simulink model "ultra"  (R2020b)
settings: Solver=FixedStepDiscrete  StartTime=0.0  StopTime=10.0  FixedStep=0.0005  RelTol=1e-3  EnableMultiTasking=on
undefined symbols (not defined in the file): acc_calmax1, acc_calmax2, acc_calmin1, acc_calmin2, akemancanshu, bre, bre_calmax, bre_calmin, ecucoder_acal, I_AN01_5K1, I_AN03_5V, I_AN04_5V, kd, ki, kp, leftmax, O_SW06_HS1A, rightmax, T_add, T_del, tiaoshi, zhiling
libraries: ec5744lib x215, canmsglib x75, simulink x10
(part 5 of 7)

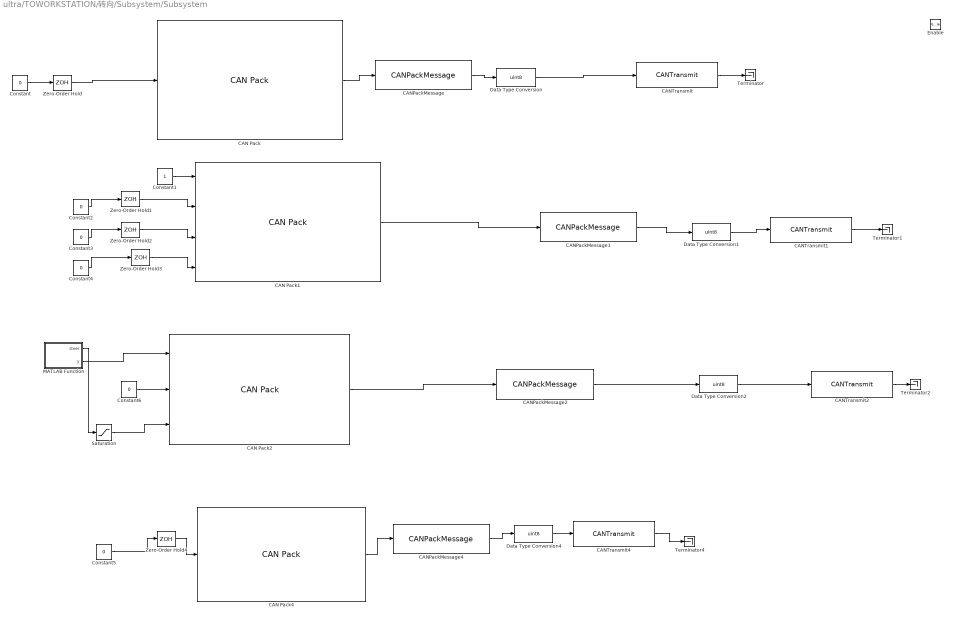
== system ultra/TOWORKSTATION/转向/Subsystem/Subsystem ==
  Enable : EnablePort
  CAN Pack : canmsglib/CAN Pack  CANdbFile=C:\Users\Liu keliang\Desktop\HRT2023\HRT23赛季刘科良\CANdbc\steering.dbc  MsgList=enable123  MsgName=enable123  MsgIDType=Standard (11-bit identifier)  MsgIdentifier=291  MsgLength=1  Remote=off  ApplyMinMax=off  BusOutput=off  SignalInfo={'enable123','0','8','LE','unsigned','Standard','0','1','0','0','255'}
      settings: SourceProductBaseCode=ME,XP,VN  DataFormat=CANdb specified signals
  CAN Pack1 : canmsglib/CAN Pack  CANdbFile=C:\Users\Liu keliang\Desktop\HRT2023\HRT23赛季刘科良\CANdbc\steering.dbc  MsgList=enable0  MsgName=enable0  MsgIDType=Standard (11-bit identifier)  MsgIdentifier=0  MsgLength=8  Remote=off  ApplyMinMax=off  BusOutput=off  SignalInfo={'enable_00','0','16','LE','unsigned','Standard','0','1','0','0','65535';'enable_00_Copy_1','16','16','LE','unsigned','Standard','0','1','0','0','65535';'enable_00_Copy_2','32','16','LE','unsigned','Standard','0','1','0','0','65535';'enable_00_Copy_3','48','16','LE','unsigned','Standard','0','1','0','0','65535'}
      settings: SourceProductBaseCode=ME,XP,VN  DataFormat=CANdb specified signals
  CAN Pack2 : canmsglib/CAN Pack  CANdbFile=C:\Users\Liu keliang\Desktop\HRT2023\HRT23赛季刘科良\CANdbc\steering.dbc  MsgList=enable401  MsgName=enable401  MsgIDType=Standard (11-bit identifier)  MsgIdentifier=1025  MsgLength=6  Remote=off  ApplyMinMax=off  BusOutput=off  SignalInfo={'enable401','0','8','LE','unsigned','Standard','0','1','0','0','255';'enable401_Copy_1','8','8','LE','unsigned','Standard','0','1','0','0','255';'enable401_Copy_2','16','32','LE','signed','Standard','0','1','0','-2147483648','2147483647'}
      settings: SourceProductBaseCode=ME,XP,VN  DataFormat=CANdb specified signals
  CAN Pack4 : canmsglib/CAN Pack  CANdbFile=C:\Users\Liu keliang\Desktop\HRT2023\HRT23赛季刘科良\CANdbc\steering.dbc  MsgList=enable80  MsgName=enable80  MsgIDType=Standard (11-bit identifier)  MsgIdentifier=128  MsgLength=1  Remote=off  ApplyMinMax=off  BusOutput=off  SignalInfo={'dingshi','0','8','LE','unsigned','Standard','0','1','0','0','255'}
      settings: SourceProductBaseCode=ME,XP,VN  DataFormat=CANdb specified signals
  CANPackMessage : ec5744lib/RapidECU_U4B/04CANCommunication/CANPackMessage  datalength=1  sampletime=-1
      settings: SourceProductName=ECUCoder for MPC5744
  CANPackMessage1 : ec5744lib/RapidECU_U4B/04CANCommunication/CANPackMessage  datalength=8  sampletime=-1
      settings: SourceProductName=ECUCoder for MPC5744
  CANPackMessage2 : ec5744lib/RapidECU_U4B/04CANCommunication/CANPackMessage  datalength=6  sampletime=-1
      settings: SourceProductName=ECUCoder for MPC5744
  CANPackMessage4 : ec5744lib/RapidECU_U4B/04CANCommunication/CANPackMessage  datalength=1  sampletime=-1
      settings: SourceProductName=ECUCoder for MPC5744
  CANTransmit : ec5744lib/RapidECU_U4B/04CANCommunication/CANTransmit  canmodule=1  canbuffer=15  canmessageid=hex2dec('123')  canmessagetype=Standard(11-bit ID)  datalength=1  sampletime=-1
      settings: SourceProductName=ECUCoder for MPC5744
  CANTransmit1 : ec5744lib/RapidECU_U4B/04CANCommunication/CANTransmit  canmodule=1  canbuffer=56  canmessageid=hex2dec('00')  canmessagetype=Standard(11-bit ID)  datalength=8  sampletime=-1
      settings: SourceProductName=ECUCoder for MPC5744
  CANTransmit2 : ec5744lib/RapidECU_U4B/04CANCommunication/CANTransmit  canmodule=1  canbuffer=57  canmessageid=hex2dec('401')  canmessagetype=Standard(11-bit ID)  datalength=6  sampletime=-1
      settings: SourceProductName=ECUCoder for MPC5744
  CANTransmit4 : ec5744lib/RapidECU_U4B/04CANCommunication/CANTransmit  canmodule=1  canbuffer=58  canmessageid=hex2dec('80')  canmessagetype=Standard(11-bit ID)  datalength=1  sampletime=-1
      settings: SourceProductName=ECUCoder for MPC5744
  Constant : Constant  Value=0  SampleTime=-1
  Constant1 : Constant  SampleTime=-1
  Constant{2..4,6} (4 alike) : Constant  Value=0
  Constant5 : Constant  Value=0  SampleTime=-1
  Data Type Conversion{,1..2,4} (4 alike) : DataTypeConversion  OutDataTypeStr=uint8
  MATLAB Function : MATLAB Function  TreatAsAtomicUnit=on
  Saturation : Saturate  UpperLimit=758000  LowerLimit=605000
  Terminator{,1..2,4} (4 alike) : Terminator
  Zero-Order Hold{,1..4} (5 alike) : ZeroOrderHold  SampleTime=-1
  wires:
  CANTransmit/1 -> Terminator/1
  Zero-Order Hold2/1 -> CAN Pack1/3
  MATLAB Function/2(y) -> CAN Pack2/1
  CAN Pack1/1 -> CANPackMessage1/1
  CANTransmit2/1 -> Terminator2/1
  CANPackMessage4/1 -> Data Type Conversion4/1
  CAN Pack2/1 -> CANPackMessage2/1
  CANTransmit1/1 -> Terminator1/1
  Constant/1 -> Zero-Order Hold/1
  Data Type Conversion1/1 -> CANTransmit1/1
  Constant6/1 -> CAN Pack2/2
  CANTransmit4/1 -> Terminator4/1
  Data Type Conversion/1 -> CANTransmit/1
  Zero-Order Hold/1 -> CAN Pack/1
  CANPackMessage2/1 -> Data Type Conversion2/1
  CANPackMessage/1 -> Data Type Conversion/1
  Data Type Conversion4/1 -> CANTransmit4/1
  Constant4/1 -> Zero-Order Hold3/1
  CAN Pack/1 -> CANPackMessage/1
  CANPackMessage1/1 -> Data Type Conversion1/1
  Constant5/1 -> Zero-Order Hold4/1
  CAN Pack4/1 -> CANPackMessage4/1
  Constant3/1 -> Zero-Order Hold2/1
  Constant2/1 -> Zero-Order Hold1/1
  Constant1/1 -> CAN Pack1/1
  Zero-Order Hold4/1 -> CAN Pack4/1
  MATLAB Function/1(steer) -> Saturation/1
  Zero-Order Hold1/1 -> CAN Pack1/2
  Data Type Conversion2/1 -> CANTransmit2/1
  Zero-Order Hold3/1 -> CAN Pack1/4
  Saturation/1 -> CAN Pack2/3

== system ultra/TOWORKSTATION/转向/Subsystem/Subsystem1 ==
  y1 : Inport
  y2 : Inport  Port=2
  Enable : EnablePort
  CAN Pack5 : canmsglib/CAN Pack  CANdbFile=C:\Users\Liu keliang\Desktop\HRT2023\HRT23赛季刘科良\CANdbc\zhuanxiangresetting.dbc  MsgList=reseting  MsgName=reseting  MsgIDType=Standard (11-bit identifier)  MsgIdentifier=1537  MsgLength=8  Remote=off  ApplyMinMax=off  BusOutput=off  SignalInfo={'reseting1','0','32','LE','unsigned','Standard','0','1','0','-Inf','Inf';'reseting2','32','32','LE','unsigned','Standard','0','1','0','-Inf','Inf'}
      settings: SourceProductBaseCode=ME,XP,VN  DataFormat=CANdb specified signals
  CANPackMessage3 : ec5744lib/RapidECU_U4B/04CANCommunication/CANPackMessage  datalength=8  sampletime=-1
      settings: SourceProductName=ECUCoder for MPC5744
  CANTransmit3 : ec5744lib/RapidECU_U4B/04CANCommunication/CANTransmit  canmodule=1  canbuffer=61  canmessageid=hex2dec('601')  canmessagetype=Standard(11-bit ID)  datalength=8  sampletime=-1
      settings: SourceProductName=ECUCoder for MPC5744
  Data Type Conversion3 : DataTypeConversion  OutDataTypeStr=uint8
  Terminator3 : Terminator
  wires:
  CAN Pack5/1 -> CANPackMessage3/1
  y1/1 -> CAN Pack5/1
  CANTransmit3/1 -> Terminator3/1
  Data Type Conversion3/1 -> CANTransmit3/1
  CANPackMessage3/1 -> Data Type Conversion3/1
  y2/1 -> CAN Pack5/2

== system ultra/TX控制器/扭矩/TEST/Subsystem ==
  Enable : EnablePort
  CAN Pack1 : canmsglib/CAN Pack  CANdbFile=C:\Users\Liu keliang\Desktop\HRT2023\HRT23赛季刘科良\CANdbc\TEST.dbc  MsgList=TEST  MsgName=TEST  MsgIDType=Standard (11-bit identifier)  MsgIdentifier=153  MsgLength=5  Remote=off  ApplyMinMax=off  BusOutput=off  SignalInfo={'M','16','8','LE','signed','Standard','0','1','0','-Inf','Inf';'X2D','32','8','LE','signed','Standard','0','1','0','-Inf','Inf';'a','0','8','LE','signed','Standard','0','1','0','-Inf','Inf';'deltv','8','8','LE','signed','Standard','0','1','0','-Inf','Inf';'niuju','24','8','LE','signed','Standard','0','1','0','-Inf','Inf'}
      settings: SourceProductBaseCode=ME,XP,VN  DataFormat=CANdb specified signals
  CANPackMessage1 : ec5744lib/RapidECU_U4B/04CANCommunication/CANPackMessage  datalength=5  sampletime=-1
      settings: SourceProductName=ECUCoder for MPC5744
  CANTransmit : ec5744lib/RapidECU_U4B/04CANCommunication/CANTransmit  canmodule=0  canbuffer=63  canmessageid=hex2dec('99')  canmessagetype=Standard(11-bit ID)  datalength=5  sampletime=-1
      settings: SourceProductName=ECUCoder for MPC5744
  Data Store Read : DataStoreRead  DataStoreName=a
  Data Store Read1 : DataStoreRead  DataStoreName=ve
  Data Store Read2 : DataStoreRead  DataStoreName=M
  Data Store Read3 : DataStoreRead  DataStoreName=acc
  Data Store Read4 : DataStoreRead  DataStoreName=dianji_velcoity_zuoqian
  Data Type Conversion1 : DataTypeConversion  OutDataTypeStr=uint8
  Terminator : Terminator
  wires:
  Data Store Read4/1 -> CAN Pack1/1
  CANTransmit/1 -> Terminator/1
  Data Store Read3/1 -> CAN Pack1/3
  CANPackMessage1/1 -> Data Type Conversion1/1
  Data Store Read2/1 -> CAN Pack1/5
  Data Type Conversion1/1 -> CANTransmit/1
  Data Store Read1/1 -> CAN Pack1/4
  Data Store Read/1 -> CAN Pack1/2
  CAN Pack1/1 -> CANPackMessage1/1

== system ultra/run/analog_input/无人意图转译/无人 ==
  Data Store Read : DataStoreRead  DataStoreName=match_model
  Data Store Write : DataStoreWrite  DataStoreName=escmax
  MATLAB Function3 : MATLAB Function  TreatAsAtomicUnit=on
  Max : MinMax  Function=max  Inputs=4
  Subsystem1 : Subsystem
  右前油压 : DataStoreWrite  DataStoreName=oral_pressure_rightfront
  右后油压 : DataStoreWrite  DataStoreName=oral_pressure_rightbehind
  左前油压 : DataStoreWrite  DataStoreName=oral_pressure_leftfront
  左后油压 : DataStoreWrite  DataStoreName=oral_pressure_leftbehind
  是否无人 : DataStoreWrite  DataStoreName=isdriveless
  期望加速度 : DataStoreWrite  DataStoreName=acc_expired
  期望纵向加速度 : Outport
  wires:
  Subsystem1/1(期望纵向加速度) -> 期望纵向加速度/1, 期望加速度/1
  Data Store Read/1 -> MATLAB Function3/1(u)
  MATLAB Function3/1(y) -> 是否无人/1
  Subsystem1/2(输出左前油压) -> Max/1, 左前油压/1
  Subsystem1/4(输出左后油压2) -> Max/3, 左后油压/1
  Subsystem1/3(输出右前油压1) -> Max/2, 右前油压/1
  Subsystem1/5(输出右后油压3) -> Max/4, 右后油压/1
  Max/1 -> Data Store Write/1

== system ultra/run/analog_input/有人/Subsystem ==
  AnalogInput : ec5744lib/RapidECU_U4B/01BasicInput/AnalogInput  channel=52:I_AN03_5V  sampletime=-1
      settings: SourceProductName=ECUCoder for MPC5744
  AnalogInput1 : ec5744lib/RapidECU_U4B/01BasicInput/AnalogInput  channel=53:I_AN04_5V  sampletime=-1
      settings: SourceProductName=ECUCoder for MPC5744
  AnalogInput2 : ec5744lib/RapidECU_U4B/01BasicInput/AnalogInput  channel=34:I_AN01_5K1  sampletime=-1
      settings: SourceProductName=ECUCoder for MPC5744
  Data Type Conversion : DataTypeConversion  OutDataTypeStr=double
  ECCalVar1 : Constant  InitFcn=ecucoder_acal;  Value=acc_calmax1  OutDataTypeStr=double  SampleTime=-1
  ECCalVar2 : Constant  InitFcn=ecucoder_acal;  Value=acc_calmin1  OutDataTypeStr=double  SampleTime=-1
  ECCalVar3 : Constant  InitFcn=ecucoder_acal;  Value=acc_calmax2  OutDataTypeStr=double  SampleTime=-1
  ECCalVar4 : Constant  InitFcn=ecucoder_acal;  Value=acc_calmin2  OutDataTypeStr=double  SampleTime=-1
  ECCalVar5 : Constant  InitFcn=ecucoder_acal;  Value=bre_calmax  OutDataTypeStr=double  SampleTime=-1
  ECCalVar6 : Constant  InitFcn=ecucoder_acal;  Value=bre_calmin  OutDataTypeStr=double  SampleTime=-1
  ECCalVar7 : Constant  InitFcn=ecucoder_acal;  Value=bre  OutDataTypeStr=double  SampleTime=-1
  FRAMEnable : ec5744lib/RapidECU_U4B/12EEModule/FRAMEnable  Commented=on  framenable=off
      settings: SourceProductName=ECUCoder for MPC5744
  MATLAB Function : MATLAB Function  TreatAsAtomicUnit=on
  MATLAB Function1 : MATLAB Function  TreatAsAtomicUnit=on
  MATLAB Function2 : MATLAB Function  TreatAsAtomicUnit=on
  MATLAB Function5 : MATLAB Function  TreatAsAtomicUnit=on
  MeaModule1 : ec5744lib/RapidECU_U4B/07Calibration/MeaModule  signal=acc_ori_line1
      settings: SourceProductName=ECUCoder for MPC5744
  MeaModule2 : ec5744lib/RapidECU_U4B/07Calibration/MeaModule  signal=acc_ori_line2
      settings: SourceProductName=ECUCoder for MPC5744
  MeaModule3 : ec5744lib/RapidECU_U4B/07Calibration/MeaModule  signal=guiyi
      settings: SourceProductName=ECUCoder for MPC5744
  MeaModule5 : ec5744lib/RapidECU_U4B/07Calibration/MeaModule  signal=bre_ori_sig
      settings: SourceProductName=ECUCoder for MPC5744
  MeaModule6 : ec5744lib/RapidECU_U4B/07Calibration/MeaModule  signal=acc_result2
      settings: SourceProductName=ECUCoder for MPC5744
  MeaModule8 : ec5744lib/RapidECU_U4B/07Calibration/MeaModule  signal=acc_result1
      settings: SourceProductName=ECUCoder for MPC5744
  MeaModule9 : ec5744lib/RapidECU_U4B/07Calibration/MeaModule  signal=bre_result
      settings: SourceProductName=ECUCoder for MPC5744
  Subsystem : Subsystem  Commented=on
  Subsystem1 : Subsystem  Commented=on
  无人制动标志位 : DataStoreRead  DataStoreName=wurenzhidongdeng
  acc : Outport
  bre : Outport  Port=2
  wires:
  AnalogInput/1 -> MeaModule1/1
  MeaModule8/1 -> MATLAB Function5/1(acc_fin_sig1)
  AnalogInput2/1 -> MeaModule5/1
  MeaModule5/1 -> MATLAB Function1/1(u)
  AnalogInput1/1 -> MeaModule2/1
  MeaModule1/1 -> MATLAB Function/1(u)
  MeaModule2/1 -> MATLAB Function2/1(u)
  MeaModule9/1 -> bre/1, MATLAB Function5/3(bre_ori_sig)
  ECCalVar3/1 -> MATLAB Function2/3(max)
  MATLAB Function2/1(y) -> MeaModule6/1
  ECCalVar1/1 -> MATLAB Function/3(max)
  ECCalVar4/1 -> MATLAB Function2/2(min)
  MATLAB Function/1(y) -> MeaModule8/1
  ECCalVar2/1 -> MATLAB Function/2(min)
  Subsystem1/1(y) -> Subsystem/Enable
  MeaModule6/1 -> Data Type Conversion/1
  Data Type Conversion/1 -> MATLAB Function5/2(acc_fin_sig2)
  ECCalVar6/1 -> MATLAB Function1/2(min)
  ECCalVar5/1 -> MATLAB Function1/3(max)
  MATLAB Function5/1(y) -> MeaModule3/1
  MeaModule3/1 -> acc/1
  ECCalVar7/1 -> MATLAB Function5/4(bre)
  无人制动标志位/1 -> MeaModule9/1

== system ultra/run/analog_input/有人/Subsystem1 ==
  note: 标定
  acc_signal : Inport
  Constant : Constant  Value=35
  Data Store Read : DataStoreRead  DataStoreName=V_Kalman
  Data Type Conversion : DataTypeConversion  OutMin=[0]  OutMax=[1]  OutDataTypeStr=double
  Divide1 : Product  Inputs=**  OutDataTypeStr=uint16
  ECCalVar : Constant  InitFcn=ecucoder_acal;  Value=T_add  OutDataTypeStr=Inherit: Inherit via back propagation  SampleTime=-1
  ECCalVar1 : Constant  InitFcn=ecucoder_acal;  Value=T_del  OutDataTypeStr=Inherit: Inherit via back propagation  SampleTime=-1
  ECCalVar2 : Constant  InitFcn=ecucoder_acal;  Value=zhiling  OutDataTypeStr=Inherit: Inherit via back propagation  SampleTime=-1
  MATLAB Function : MATLAB Function  TreatAsAtomicUnit=on
  MATLAB Function1 : MATLAB Function  TreatAsAtomicUnit=on
  Saturation3 : Saturate  UpperLimit=2100  LowerLimit=0
  Saturation4 : Saturate  UpperLimit=1  LowerLimit=0
  Sum : Sum  Inputs=|++-
  Sum1 : Sum  Inputs=+--
  TP : Outport
  wires:
  Data Type Conversion/1 -> Saturation4/1
  acc_signal/1 -> Data Type Conversion/1
  Saturation4/1 -> Divide1/2
  Sum/1 -> Divide1/1
  ECCalVar1/1 -> Sum/3
  ECCalVar/1 -> Sum/1
  Saturation3/1 -> Sum/2
  Data Store Read/1 -> MATLAB Function/1(v)
  MATLAB Function/1(T) -> Saturation3/1
  Divide1/1 -> Sum1/1
  Constant/1 -> Sum1/2
  Sum1/1 -> MATLAB Function1/1(T)
  MATLAB Function1/1(TP) -> TP/1
  ECCalVar2/1 -> Sum1/3

== system ultra/run/ctrl/Subsystem1/control_strategy ==
  TP : Inport
  Data Store Read1 : DataStoreRead  DataStoreName=workstation_steering
  Data Store Read2 : DataStoreRead  DataStoreName=slipyouhou
  Data Store Read4 : DataStoreRead  DataStoreName=workstation_steering
  Data Store Read5 : DataStoreRead  DataStoreName=slipzuohou
  Data Store Read6 : DataStoreRead  DataStoreName=slipyuoqian
  Data Store Read7 : DataStoreRead  DataStoreName=slipzuoqian
  E,H : MATLAB Function  Commented=on  TreatAsAtomicUnit=on
  MATLAB Function : MATLAB Function  Commented=on  TreatAsAtomicUnit=on
  MATLAB Function1 : MATLAB Function  TreatAsAtomicUnit=on
  MATLAB Function2 : MATLAB Function  Commented=on  TreatAsAtomicUnit=on
  MATLAB Function3 : MATLAB Function  TreatAsAtomicUnit=on
  MPC : MATLAB Function  Commented=on  TreatAsAtomicUnit=on
  Subsystem : Subsystem  Commented=on
  Switch{,1..3} (4 alike) : Switch  Criteria=u2 > Threshold
  差速 : Subsystem
  滑模控制 : MATLAB Function  TreatAsAtomicUnit=on
  限滑 : Subsystem
  youhou : Outport
  youqian : Outport  Port=2
  zuohou : Outport  Port=3
  zuoqian : Outport  Port=4
  wires:
  TP/1 -> 差速/1(u), 限滑/1(In1)
  Data Store Read4/1 -> MATLAB Function1/1(angle)
  MATLAB Function1/1(y) -> Switch2/2, Switch3/2, Switch1/2, Switch/2
  限滑/1(youhou) -> Switch/3
  限滑/2(youqian) -> Switch1/3
  限滑/3(zuohou) -> Switch2/3
  限滑/4(zuoqian) -> Switch3/3
  MATLAB Function2/1(A) -> E,H/1(A)
  MATLAB Function2/2(B) -> E,H/2(B)
  MATLAB Function2/3(Q) -> E,H/3(Q)
  MATLAB Function2/4(R) -> E,H/4(R)
  MATLAB Function2/5(F) -> E,H/5(F)
  MATLAB Function2/6(N) -> E,H/6(N)
  差速/1(youhou) -> Switch/1
  差速/2(youqian) -> Switch1/1
  差速/3(zuohou) -> Switch2/1
  差速/4(zuoqian) -> Switch3/1
  Data Store Read1/1 -> MATLAB Function3/1(angle)
  MATLAB Function3/1(y) -> 差速/Enable
  Data Store Read7/1 -> 滑模控制/1(slip_ratio_fl)
  Switch/1 -> 滑模控制/8(driver_torque_cmd_rr)
  Data Store Read2/1 -> 滑模控制/4(slip_ratio_rr)
  Data Store Read6/1 -> 滑模控制/2(slip_ratio_fr)
  Switch3/1 -> 滑模控制/5(driver_torque_cmd_fl)
  Data Store Read5/1 -> 滑模控制/3(slip_ratio_rl)
  Switch1/1 -> 滑模控制/6(driver_torque_cmd_fr)
  Switch2/1 -> 滑模控制/7(driver_torque_cmd_rl)
  滑模控制/4(torque_cmd_rr) -> youhou/1
  滑模控制/2(torque_cmd_fr) -> youqian/1
  滑模控制/3(torque_cmd_rl) -> zuohou/1
  滑模控制/1(torque_cmd_fl) -> zuoqian/1

== system ultra/RX/工作站/Subsystem1/Subsystem1/Subsystem ==
  ID : Inport
  msg : Inport  Port=2
  CAN Unpack : canmsglib/CAN Unpack  CANdbFile=C:\Users\Liu keliang\Desktop\HRT2023\HRT23赛季刘科良\CANdbc\INSWORKSTATION.dbc  MsgList=ins  MsgName=ins  MsgIDType=Standard (11-bit identifier)  MsgIdentifier=33  MsgLength=8  SignalInfo={'Vx','32','16','LE','unsigned','Standard','0','1','0','0','65535';'Vy','48','16','LE','unsigned','Standard','0','1','0','0','65535';'ax','0','8','LE','signed','Standard','0','1','0','-128','127';'ay','8','16','LE','signed','Standard','0','1','0','-32768','32767';'az','24','8','LE','signed','Standard','0','1','0','-128','127'}  IDPort=off  TimestampPort=off  ErrorPort=off  RemotePort=off  LengthPort=off  StatusPort=off  ApplyMinMax=off
      settings: SourceProductBaseCode=ME,XP,VN  DataFormat=CANdb specified signals
  CANUnPackMessage : ec5744lib/RapidECU_U4B/04CANCommunication/CANUnPackMessage  datalength=8  canmessagetype=Standard(11-bit ID)  sampletime=-1
      settings: SourceProductName=ECUCoder for MPC5744
  Data Store Write : DataStoreWrite  DataStoreName=guandaovy
  wires:
  msg/1 -> CANUnPackMessage/2
  CANUnPackMessage/1 -> CAN Unpack/1
  ID/1 -> CANUnPackMessage/1
  CAN Unpack/2 -> Data Store Write/1

== system ultra/RX/工作站/Subsystem3/Subsystem/Subsystem ==
  Data Store Read : DataStoreRead  DataStoreName=CANOK_20
  Delay : Delay  DelayLength=1
  Delay1 : Delay
  Delay10 : Delay  DelayLength=11
  Delay11 : Delay  DelayLength=12
  Delay12 : Delay  DelayLength=13
  Delay13 : Delay  DelayLength=14
  Delay14 : Delay  DelayLength=15
  Delay15 : Delay  DelayLength=16
  Delay16 : Delay  DelayLength=17
  Delay17 : Delay  DelayLength=25
  Delay18 : Delay  DelayLength=18
  Delay19 : Delay  DelayLength=19
  Delay2 : Delay  DelayLength=3
  Delay20 : Delay  DelayLength=20
  Delay21 : Delay  DelayLength=21
  Delay22 : Delay  DelayLength=22
  Delay23 : Delay  DelayLength=26
  Delay24 : Delay  DelayLength=24
  Delay25 : Delay  DelayLength=27
  Delay3 : Delay  DelayLength=4
  Delay4 : Delay  DelayLength=5
  Delay5 : Delay  DelayLength=6
  Delay6 : Delay  DelayLength=7
  Delay7 : Delay  DelayLength=8
  Delay8 : Delay  DelayLength=9
  Delay9 : Delay  DelayLength=10
  OR : Logic  Operator=OR  Inputs=27  IconShape=distinctive  AllPortsSameDT=off  OutDataTypeStr=boolean
  Out1 : Outport
  wires:
  Delay2/1 -> OR/2
  Delay/1 -> OR/4
  Data Store Read/1 -> Delay23/1, Delay25/1, Delay17/1, Delay24/1, Delay22/1, Delay21/1, Delay20/1, Delay19/1, Delay18/1, Delay16/1, Delay15/1, Delay14/1, Delay13/1, Delay12/1, Delay11/1, Delay10/1, Delay8/1, Delay6/1, Delay5/1, Delay7/1, Delay9/1, OR/5, Delay3/1, Delay2/1, Delay1/1, Delay/1, Delay4/1
  Delay5/1 -> OR/7
  Delay1/1 -> OR/3
  Delay9/1 -> OR/11
  Delay7/1 -> OR/9
  Delay3/1 -> OR/1
  Delay8/1 -> OR/8
  Delay6/1 -> OR/6
  Delay4/1 -> OR/10
  OR/1 -> Out1/1
  Delay10/1 -> OR/12
  Delay11/1 -> OR/13
  Delay12/1 -> OR/14
  Delay13/1 -> OR/15
  Delay14/1 -> OR/16
  Delay15/1 -> OR/17
  Delay16/1 -> OR/18
  Delay18/1 -> OR/19
  Delay19/1 -> OR/20
  Delay20/1 -> OR/21
  Delay21/1 -> OR/22
  Delay22/1 -> OR/23
  Delay24/1 -> OR/24
  Delay17/1 -> OR/25
  Delay23/1 -> OR/27
  Delay25/1 -> OR/26

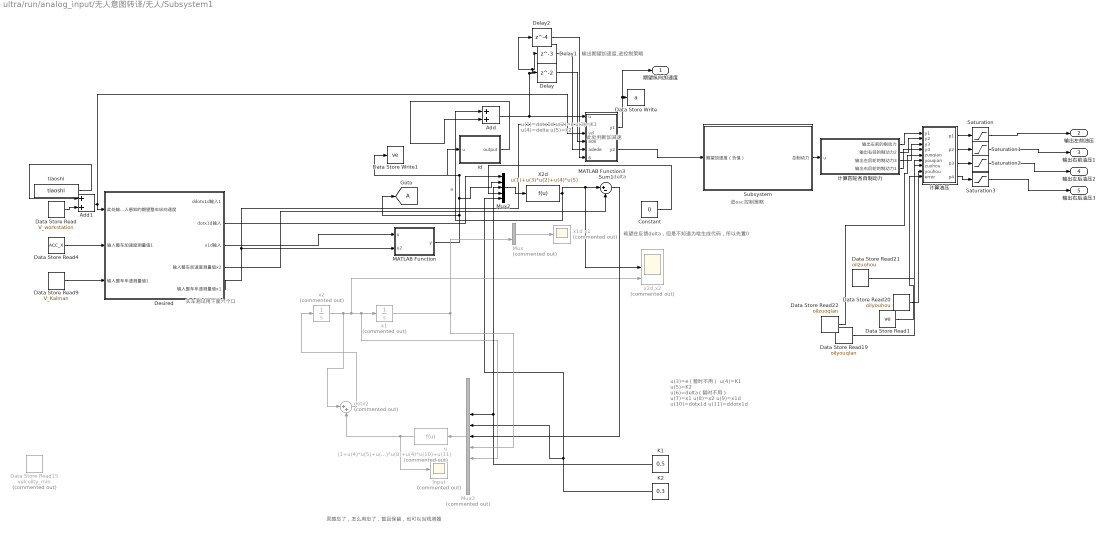
== system ultra/run/analog_input/无人意图转译/无人/Subsystem1 ==
  note: 希望在反馈delta，但是不知道为啥生成代码，所以先置0
  note: 灵感忘了，怎么用忘了，暂且保留，也可以当观测器
  note: 输出期望加速度,进控制策略
  note: 进esc控制策略
  note: u(3)=e（暂时不用）
      | u(4)=K1
      | u(5)=K2
      | u(6)=delta（暂时不用）
      | u(7)=x1
      | u(8)=x2
      | u(9)=x1d
      | u(10)=dotx1d
      | u(11)=ddotx1d
  note: delta
  note: e
  note: 此处判断加减速
  note: 实车测试用下面六个口
  note: u(1)=dotx1d
      | u(2)=e
      | u(3)=K1
      | u(4)=delta
      | u(5)=k2
  Add : Sum
  Add1 : Sum
  Constant : Constant  Value=0
  Data Store Read : DataStoreRead  DataStoreName=V_workstation
  Data Store Read1 : DataStoreRead  DataStoreName=ve
  Data Store Read15 : DataStoreRead  Commented=on  DataStoreName=velcolity_min
  Data Store Read19 : DataStoreRead  DataStoreName=oilyouqian
  Data Store Read20 : DataStoreRead  DataStoreName=oilyouhou
  Data Store Read21 : DataStoreRead  DataStoreName=oilzuohou
  Data Store Read22 : DataStoreRead  DataStoreName=oilzuoqian
  Data Store Read4 : DataStoreRead  DataStoreName=ACC_X
  Data Store Read9 : DataStoreRead  DataStoreName=V_Kalman
  Data Store Write : DataStoreWrite  DataStoreName=a
  Data Store Write1 : DataStoreWrite  DataStoreName=ve
  Delay : Delay
  Delay1 : Delay  DelayLength=3
  Delay2 : Delay  DelayLength=4
  Desired : Subsystem
  "Input " : Scope  Commented=on
  K1 : Constant  Value=0.5
  K2 : Constant  Value=0.3
  MATLAB Function : MATLAB Function  TreatAsAtomicUnit=on
  MATLAB Function3 : MATLAB Function  TreatAsAtomicUnit=on
  Mux : Mux  Commented=on  Inputs=2
  Mux2 : Mux  Inputs=5
  Mux3 : Mux  Commented=on  Inputs=11
  Saturation{,1..3} (4 alike) : Saturate  UpperLimit=3500  LowerLimit=0
  Subsystem : Subsystem
  Sum1 : Sum  Inputs=|+-
  X2d : Fcn  Expr=u(1)+u(3)*u(2)+u(4)*u(5)
  dotx2 : Sum  Commented=on  Inputs=|++
  id : MATLAB Function  TreatAsAtomicUnit=on
  tiaoshi : Constant  InitFcn=ecucoder_acal;  Value=tiaoshi  OutDataTypeStr=double  SampleTime=-1
  u : Fcn  Commented=on  Expr=(1+u(4)*u(5)+u(5))*u(9)-(1+u(4)*u(5))*u(7)-(u(4)+u(5)-1)*u(8)+u(4)*u(10)+u(11)
  x1 : Integrator  Commented=on
  x1d x1 : Scope  Commented=on
  x2 : Integrator  Commented=on  UpperSaturationLimit=10  ZeroCross=off
  x2d,x2 : Scope  Commented=on  NumInputPorts=3
  计算四轮各自制动力 : Subsystem
  计算油压 : MATLAB Function  TreatAsAtomicUnit=on
  期望纵向加速度 : Outport
  输出左前油压 : Outport  Port=2
  输出右前油压1 : Outport  Port=3
  输出左后油压2 : Outport  Port=4
  输出右后油压3 : Outport  Port=5
  tag scope: A=global
  wires:
  K2/1 -> Mux2/5, Mux3/5
  计算油压/1(p1) -> Saturation/1
  MATLAB Function/1(y) -> Data Store Write1/1, id/1(u), Mux2/2, [A]
  Desired/4(输入整车加速度测量值x2) -> Sum1/2
  x2/1 -> dotx2/1, x2d,x2/3, x1/1, Mux3/8
  Sum1/1 -> Mux3/6
  计算油压/2(p2) -> Saturation1/1
  MATLAB Function3/2(y2) -> Subsystem/1(期望加速度（负值）)
  计算四轮各自制动力/1(输出左前的制动力) -> 计算油压/1(y1)
  Saturation3/1 -> 输出右后油压3/1
  Mux/1 -> x1d x1/1
  u/1 -> dotx2/2, "Input "/1
  Saturation2/1 -> 输出左后油压2/1
  Saturation1/1 -> 输出右前油压1/1
  计算油压/3(p3) -> Saturation2/1
  计算四轮各自制动力/3(输出左后轮的制动力3) -> 计算油压/3(y3)
  计算油压/4(p4) -> Saturation3/1
  Saturation/1 -> 输出左前油压/1
  计算四轮各自制动力/4(输出右后轮的制动力1) -> 计算油压/4(y4)
  Subsystem/1(总制动力) -> 计算四轮各自制动力/1(u)
  K1/1 -> Mux2/3, Mux3/4
  计算四轮各自制动力/2(输出右前的制动力2) -> 计算油压/2(y2)
  dotx2/1 -> x2/1
  Mux2/1 -> X2d/1
  Mux3/1 -> u/1
  x1/1 -> Mux/2, Mux3/7
  Data Store Read9/1 -> Desired/3(输入整车车速测量值1)
  Data Store Read4/1 -> Desired/2(输入整车加速度测量值1)
  X2d/1 -> x2d,x2/2, Sum1/1, Add/1
  Constant/1 -> Mux2/4
  MATLAB Function3/1(y1) -> Data Store Write/1, 期望纵向加速度/1
  Desired/3(x1d输入) -> MATLAB Function/1(u)
  Desired/2(dotx1d输入) -> Mux2/1
  tiaoshi/1 -> Add1/1
  Data Store Read/1 -> Add1/2
  Add1/1 -> Desired/1(此处输入感知的期望整车纵向速度), MATLAB Function3/3(vd)
  Desired/5(输入整车车速测量值x1) -> MATLAB Function/2(u2), MATLAB Function3/2(v)
  Add/1 -> Delay1/1, Delay2/1, Delay/1, MATLAB Function3/1(u)
  Delay/1 -> MATLAB Function3/4(ade)
  Delay1/1 -> MATLAB Function3/5(adede)
  Delay2/1 -> MATLAB Function3/6(adedede)
  id/1(output) -> Add/2
  Data Store Read20/1 -> 计算油压/8(youhou)
  Data Store Read21/1 -> 计算油压/7(zuohou)
  Data Store Read22/1 -> 计算油压/5(zuoqian)
  Data Store Read19/1 -> 计算油压/6(youqian)
  Data Store Read1/1 -> 计算油压/9(error)

== system ultra/run/analog_input/有人/Subsystem/Subsystem ==
  Enable : EnablePort
  Data Type Conversion{,1,4..7} (6 alike) : DataTypeConversion  OutDataTypeStr=single
  ECCalVar1 : Constant  InitFcn=ecucoder_acal;  Value=acc_calmax1  OutDataTypeStr=double  SampleTime=-1
  ECCalVar2 : Constant  InitFcn=ecucoder_acal;  Value=acc_calmin1  OutDataTypeStr=double  SampleTime=-1
  ECCalVar3 : Constant  InitFcn=ecucoder_acal;  Value=acc_calmax2  OutDataTypeStr=double  SampleTime=-1
  ECCalVar4 : Constant  InitFcn=ecucoder_acal;  Value=acc_calmin2  OutDataTypeStr=double  SampleTime=-1
  ECCalVar5 : Constant  InitFcn=ecucoder_acal;  Value=bre_calmax  OutDataTypeStr=double  SampleTime=-1
  ECCalVar6 : Constant  InitFcn=ecucoder_acal;  Value=bre_calmin  OutDataTypeStr=double  SampleTime=-1
  FRAMEnable : ec5744lib/RapidECU_U4B/12EEModule/FRAMEnable  framenable=off
      settings: SourceProductName=ECUCoder for MPC5744
  FRAMWrite1 : ec5744lib/RapidECU_U4B/12EEModule/FRAMWrite  buffer=6  sampletime=-1
      settings: SourceProductName=ECUCoder for MPC5744
  FRAMWrite2 : ec5744lib/RapidECU_U4B/12EEModule/FRAMWrite  buffer=4  sampletime=-1
      settings: SourceProductName=ECUCoder for MPC5744
  FRAMWrite3 : ec5744lib/RapidECU_U4B/12EEModule/FRAMWrite  buffer=5  sampletime=-1
      settings: SourceProductName=ECUCoder for MPC5744
  FRAMWrite4 : ec5744lib/RapidECU_U4B/12EEModule/FRAMWrite  buffer=7  sampletime=-1
      settings: SourceProductName=ECUCoder for MPC5744
  FRAMWrite5 : ec5744lib/RapidECU_U4B/12EEModule/FRAMWrite  buffer=8  sampletime=-1
      settings: SourceProductName=ECUCoder for MPC5744
  FRAMWrite6 : ec5744lib/RapidECU_U4B/12EEModule/FRAMWrite  buffer=9  sampletime=-1
      settings: SourceProductName=ECUCoder for MPC5744
  wires:
  ECCalVar2/1 -> Data Type Conversion/1
  Data Type Conversion/1 -> FRAMWrite5/1
  ECCalVar5/1 -> Data Type Conversion7/1
  Data Type Conversion7/1 -> FRAMWrite3/1
  Data Type Conversion6/1 -> FRAMWrite2/1
  ECCalVar6/1 -> Data Type Conversion6/1
  ECCalVar3/1 -> Data Type Conversion5/1
  Data Type Conversion5/1 -> FRAMWrite4/1
  ECCalVar4/1 -> Data Type Conversion4/1
  Data Type Conversion4/1 -> FRAMWrite1/1
  ECCalVar1/1 -> Data Type Conversion1/1
  Data Type Conversion1/1 -> FRAMWrite6/1

== system ultra/run/analog_input/有人/Subsystem/Subsystem1 ==
  ECCalVar1 : Constant  InitFcn=ecucoder_acal;  Value=acc_calmax1  OutDataTypeStr=double  SampleTime=-1
  ECCalVar2 : Constant  InitFcn=ecucoder_acal;  Value=acc_calmin1  OutDataTypeStr=double  SampleTime=-1
  ECCalVar3 : Constant  InitFcn=ecucoder_acal;  Value=acc_calmax2  OutDataTypeStr=double  SampleTime=-1
  ECCalVar4 : Constant  InitFcn=ecucoder_acal;  Value=acc_calmin2  OutDataTypeStr=double  SampleTime=-1
  ECCalVar5 : Constant  InitFcn=ecucoder_acal;  Value=bre_calmax  OutDataTypeStr=double  SampleTime=-1
  ECCalVar6 : Constant  InitFcn=ecucoder_acal;  Value=bre_calmin  OutDataTypeStr=double  SampleTime=-1
  MATLAB Function : MATLAB Function  TreatAsAtomicUnit=on
  Max : MinMax  Function=max  Inputs=6
  y : Outport
  wires:
  ECCalVar3/1 -> Max/4
  ECCalVar2/1 -> Max/1
  ECCalVar4/1 -> Max/3
  ECCalVar5/1 -> Max/6
  ECCalVar1/1 -> Max/2
  ECCalVar6/1 -> Max/5
  Max/1 -> MATLAB Function/1(u)
  MATLAB Function/1(y) -> y/1

== system ultra/run/ctrl/Subsystem1/control_strategy/Subsystem ==
  alpha : Inport
  beta : Inport  Port=2
  -1~1 : Saturate  Commented=on  UpperLimit=1  LowerLimit=-1
  0~5 : Saturate  Commented=on  UpperLimit=5  LowerLimit=0
  Mux : Mux  Commented=on  Inputs=3
  Mux1 : Mux  Commented=on  Inputs=5
  Mux2 : Mux  Commented=on  Inputs=5
  Rules : Subsystem  Commented=on
  Scope alpha : Scope  Commented=on
  Scope beta : Scope  Commented=on
  Scope delta : Scope  Commented=on
  Scope delta sets : Scope  Commented=on
  a1 : Constant  Commented=on  Value=1.2
  a2 : Constant  Commented=on  Value=2.4
  alpha test : simulink/Sources/Ramp  Commented=on  slope=0.1  start=0  InitialOutput=-0.5
  b1 : Constant  Commented=on  Value=-0.5
  b2 : Constant  Commented=on  Value=0
  b3 : Constant  Commented=on  Value=0.5
  beta test : simulink/Sources/Ramp  Commented=on  slope=0.1  start=0  InitialOutput=-1.5
  d1 : Constant  Commented=on  Value=-0.5
  d2 : Constant  Commented=on  Value=0
  d3 : Constant  Commented=on  Value=0.5
  defuzzification : MATLAB Function  Commented=on  TreatAsAtomicUnit=on
  α sets : MATLAB Function  Commented=on  TreatAsAtomicUnit=on
  β sets : MATLAB Function  Commented=on  TreatAsAtomicUnit=on
  delta : Outport  VectorParamsAs1DForOutWhenUnconnected=off
  wires:
  defuzzification/1(delta) -> delta/1, Scope delta/1  "delta"
  Rules/3(do) -> Mux2/3, defuzzification/3(do)
  Rules/5(dpb) -> Mux2/5, defuzzification/5(dpb)
  beta/1 -> -1~1/1
  b3/1 -> β sets/4(b3)
  α sets/1(as) -> Mux/1, Rules/1(as)  "as"
  β sets/3(bo) -> Mux1/3, Rules/6(bo)  "bo"
  d2/1 -> defuzzification/7(d2)
  Rules/4(dps) -> Mux2/4, defuzzification/4(dps)
  β sets/1(bnb) -> Mux1/1, Rules/4(bnb)  "bnb"
  Rules/2(dns) -> Mux2/2, defuzzification/2(dns)
  Mux/1 -> Scope alpha/1
  d1/1 -> defuzzification/6(d1)
  Mux2/1 -> Scope delta sets/1
  β sets/2(bns) -> Mux1/2, Rules/5(bns)  "bns"
  β sets/5(bpb) -> Mux1/5, Rules/8(bpb)  "bpb"
  0~5/1 -> α sets/1(alpha)
  a1/1 -> α sets/2(a1)
  alpha/1 -> 0~5/1
  β sets/4(bps) -> Mux1/4, Rules/7(bps)  "bps"
  Rules/1(dnb) -> Mux2/1, defuzzification/1(dnb)
  Mux1/1 -> Scope beta/1
  -1~1/1 -> β sets/1(beta)
  b2/1 -> β sets/3(b2)
  b1/1 -> β sets/2(b1)
  a2/1 -> α sets/3(a2)
  α sets/2(am) -> Mux/2, Rules/2(am)
  d3/1 -> defuzzification/8(d3)
  α sets/3(ab) -> Mux/3, Rules/3(ab)  "ab"

== system ultra/run/ctrl/Subsystem1/control_strategy/差速 ==
  u : Inport
  Enable : EnablePort
  MATLAB Function3 : MATLAB Function  TreatAsAtomicUnit=on
  差速 : Subsystem
  youhou : Outport
  youqian : Outport  Port=2
  zuohou : Outport  Port=3
  zuoqian : Outport  Port=4
  wires:
  MATLAB Function3/3(zuohou) -> zuohou/1
  MATLAB Function3/4(zuoqian) -> zuoqian/1
  差速/1(M) -> MATLAB Function3/2(M)
  MATLAB Function3/2(youqian) -> youqian/1
  u/1 -> MATLAB Function3/1(u)
  MATLAB Function3/1(youhou) -> youhou/1

== system ultra/run/ctrl/Subsystem1/control_strategy/限滑 ==
  In1 : Inport
  MATLAB Function : MATLAB Function  Commented=on  TreatAsAtomicUnit=on
  MPC : Subsystem
  PID限滑 : Subsystem
  Subsystem1 : Subsystem
  youhou : Outport
  youqian : Outport  Port=2
  zuohou : Outport  Port=3
  zuoqian : Outport  Port=4
  wires:
  MPC/2(左后) -> Subsystem1/8(mpc)
  PID限滑/2(throttle_youqian) -> Subsystem1/6(throttle_youqian)
  In1/1 -> PID限滑/1(u), Subsystem1/10(In7), MPC/4(左前in), Subsystem1/1(TP), MPC/1(右后in), Subsystem1/7(u), MPC/2(左后in), Subsystem1/4(In4), MPC/3(右前in)
  MPC/3(右前) -> Subsystem1/5(右前)
  PID限滑/4(throttle_zuoqian) -> Subsystem1/12(throttle_zuoqian)
  PID限滑/3(throttle_zuohou) -> Subsystem1/9(pid)
  MPC/1(右后) -> Subsystem1/2(右后)
  MPC/4(左前) -> Subsystem1/11(左前)
  PID限滑/1(throttle_youhou) -> Subsystem1/3(throttle_youhou)
  Subsystem1/1(youhou) -> youhou/1
  Subsystem1/4(zuoqian) -> zuoqian/1
  Subsystem1/3(zuohou) -> zuohou/1
  Subsystem1/2(youqian) -> youqian/1

== system ultra/run/analog_input/无人意图转译/无人/Subsystem1/Desired ==
  此处输入感知的期望整车纵向速度 : Inport
  输入整车加速度测量值1 : Inport  Port=2
  输入整车车速测量值1 : Inport  Port=3
  Data Store Read3 : DataStoreRead  DataStoreName=match_model
  Data Store Write : DataStoreWrite  DataStoreName=acc
  MATLAB Function : MATLAB Function  TreatAsAtomicUnit=on
  MATLAB Function1 : MATLAB Function  Commented=on  TreatAsAtomicUnit=on
  MATLAB Function2 : MATLAB Function  TreatAsAtomicUnit=on
  Subsystem : Subsystem
  Subsystem1 : Subsystem
  ddotx1d输入1 : Outport
  dotx1d输入 : Outport  Port=2
  x1d输入 : Outport  Port=3
  输入整车加速度测量值x2 : Outport  Port=4
  输入整车车速测量值x1 : Outport  Port=5
  wires:
  此处输入感知的期望整车纵向速度/1 -> MATLAB Function2/7(v1), Subsystem1/1(y), MATLAB Function/1(u)
  输入整车加速度测量值1/1 -> 输入整车加速度测量值x2/1
  MATLAB Function1/1(y) -> ddotx1d输入1/1
  MATLAB Function/1(y) -> MATLAB Function2/1(u1), Subsystem/1(y)
  MATLAB Function2/1(y) -> MATLAB Function1/1(u), dotx1d输入/1, Data Store Write/1
  Subsystem/1(u2) -> MATLAB Function2/2(u2)
  Subsystem/2(u3) -> MATLAB Function2/3(u3)
  Subsystem/3(u4) -> MATLAB Function2/4(u4)
  Subsystem/4(u5) -> MATLAB Function2/5(u5)
  输入整车车速测量值1/1 -> 输入整车车速测量值x1/1
  Data Store Read3/1 -> MATLAB Function2/6(model)
  Subsystem1/1(u2) -> MATLAB Function2/8(v2)
  Subsystem1/2(u3) -> MATLAB Function2/9(v3)
  Subsystem1/3(u4) -> MATLAB Function2/10(v4)
  Subsystem1/4(u5) -> MATLAB Function2/11(v5)
  MATLAB Function2/2(V) -> x1d输入/1

== system ultra/run/analog_input/无人意图转译/无人/Subsystem1/Subsystem ==
  note: 反馈系数，得调一下
  期望加速度（负值） : Inport
  Abs : Abs
  Abs1 : Abs
  Product : Product
  Sum : Sum  Inputs=|++
  pid_function : Subsystem
  整车质量 : Constant  Value=230
  总制动力 : Outport
  wires:
  期望加速度（负值）/1 -> pid_function/2(期望加速度（负值）), Abs/1
  Abs/1 -> Product/2
  整车质量/1 -> Product/1
  Product/1 -> Sum/1
  [A] -> pid_function/1(u)
  Sum/1 -> 总制动力/1
  pid_function/1(output) -> Abs1/1
  Abs1/1 -> Sum/2

== system ultra/run/analog_input/无人意图转译/无人/Subsystem1/计算四轮各自制动力 ==
  u : Inport
  Data Store Read : DataStoreRead  DataStoreName=M_expire
  MATLAB Function : MATLAB Function  TreatAsAtomicUnit=on
  输出左前的制动力 : Outport
  输出右前的制动力2 : Outport  Port=2
  输出左后轮的制动力3 : Outport  Port=3
  输出右后轮的制动力1 : Outport  Port=4
  wires:
  u/1 -> MATLAB Function/1(u)
  MATLAB Function/1(y1) -> 输出左前的制动力/1
  MATLAB Function/2(y2) -> 输出右前的制动力2/1
  MATLAB Function/3(y3) -> 输出左后轮的制动力3/1
  MATLAB Function/4(y4) -> 输出右后轮的制动力1/1
  Data Store Read/1 -> MATLAB Function/2(deltaM)

== system ultra/run/ctrl/Subsystem1/control_strategy/Subsystem/Rules ==
  as : Inport
  am : Inport  Port=2
  ab : Inport  Port=3
  bnb : Inport  Port=4
  bns : Inport  Port=5
  bo : Inport  Port=6
  bps : Inport  Port=7
  bpb : Inport  Port=8
  DNB : MinMax  Function=max
  DNS : MinMax  Function=max  Inputs=3
  DO : MinMax  Function=max  Inputs=3
  DPB : MinMax  Function=max  Inputs=4
  DPS : MinMax  Function=max  Inputs=4
  Min(AB,BNB) : MinMax  Inputs=2
  Min(AB,BNS) : MinMax  Inputs=2
  Min(AB,BO) : MinMax  Inputs=2
  Min(AB,BPB) : MinMax  Inputs=2
  Min(AB,BPS) : MinMax  Inputs=2
  Min(AM,BNB) : MinMax  Inputs=2
  Min(AM,BNS) : MinMax  Inputs=2
  Min(AM,BO) : MinMax  Inputs=2
  Min(AM,BPB) : MinMax  Inputs=2
  Min(AM,BPS) : MinMax  Inputs=2
  Min(AS,BNB) : MinMax  Inputs=2
  Min(AS,BNS) : MinMax  Inputs=2
  Min(AS,BO) : MinMax  Inputs=2
  Min(AS,BPB) : MinMax  Inputs=2
  Min(AS,BPS) : MinMax  Inputs=2
  dnb : Outport  VectorParamsAs1DForOutWhenUnconnected=off
  dns : Outport  Port=2  VectorParamsAs1DForOutWhenUnconnected=off
  do : Outport  Port=3  VectorParamsAs1DForOutWhenUnconnected=off
  dps : Outport  Port=4  VectorParamsAs1DForOutWhenUnconnected=off
  dpb : Outport  Port=5  VectorParamsAs1DForOutWhenUnconnected=off
  wires:
  Min(AS,BNS)/1 -> DNS/1
  Min(AB,BNB)/1 -> DNS/3
  bps/1 -> Min(AB,BPS)/2, Min(AM,BPS)/2, Min(AS,BPS)/2
  bo/1 -> Min(AB,BO)/2, Min(AM,BO)/2, Min(AS,BO)/2
  bpb/1 -> Min(AB,BPB)/2, Min(AM,BPB)/2, Min(AS,BPB)/2
  as/1 -> Min(AS,BPB)/1, Min(AS,BPS)/1, Min(AS,BO)/1, Min(AS,BNS)/1, Min(AS,BNB)/1
  Min(AS,BNB)/1 -> DNB/1
  Min(AS,BPB)/1 -> DPB/1
  bns/1 -> Min(AB,BNS)/2, Min(AM,BNS)/2, Min(AS,BNS)/2
  Min(AB,BNS)/1 -> DO/3
  ab/1 -> Min(AB,BPB)/1, Min(AB,BPS)/1, Min(AB,BO)/1, Min(AB,BNS)/1, Min(AB,BNB)/1
  bnb/1 -> Min(AM,BNB)/2, Min(AS,BNB)/2, Min(AB,BNB)/2
  Min(AM,BO)/1 -> DPS/3
  am/1 -> Min(AM,BPB)/1, Min(AM,BPS)/1, Min(AM,BO)/1, Min(AM,BNS)/1, Min(AM,BNB)/1
  Min(AB,BPB)/1 -> DPB/3
  Min(AM,BNB)/1 -> DNS/2
  Min(AS,BPS)/1 -> DPS/1
  Min(AM,BPS)/1 -> DPS/2
  Min(AM,BNS)/1 -> DO/2
  Min(AB,BO)/1 -> DPS/4
  Min(AS,BO)/1 -> DO/1
  Min(AM,BPB)/1 -> DPB/2
  Min(AB,BPS)/1 -> DPB/4
  DO/1 -> do/1
  DNB/1 -> dnb/1
  DNS/1 -> dns/1
  DPS/1 -> dps/1
  DPB/1 -> dpb/1

== system ultra/run/ctrl/Subsystem1/control_strategy/差速/差速 ==
  Data Store Read : DataStoreRead  DataStoreName=workstation_steering
  Data Store Read1 : DataStoreRead  DataStoreName=V_Kalman
  Data Store Read2 : DataStoreRead  DataStoreName=A_cexiang
  Data Store Read3 : DataStoreRead  DataStoreName=ACC_Z
  Data Store Read4 : DataStoreRead  Commented=on  DataStoreName=dianji_velcoity_zuoqian
  Data Store Read5 : DataStoreRead  Commented=on  DataStoreName=dianji_velcoity_youqian
  Data Store Read6 : DataStoreRead  Commented=on  DataStoreName=dianji_velcoity_zuohou
  Data Store Read7 : DataStoreRead  Commented=on  DataStoreName=dianji_velcoity_youhou
  Data Store Read8 : DataStoreRead  DataStoreName=workstation_steering
  Data Store Write1 : DataStoreWrite  DataStoreName=Vzuoqian
  Data Store Write2 : DataStoreWrite  DataStoreName=Vyouqian
  Data Store Write3 : DataStoreWrite  DataStoreName=Vzuohou
  Data Store Write4 : DataStoreWrite  DataStoreName=Vyouhou
  LQR差速 : MATLAB Function  TreatAsAtomicUnit=on
  MATLAB Function : MATLAB Function  TreatAsAtomicUnit=on
  Product : Product
  Sum : Sum  Inputs=|+-
  pid : MATLAB Function  Commented=on  TreatAsAtomicUnit=on
  pid1 : MATLAB Function  Commented=on  TreatAsAtomicUnit=on
  pid2 : MATLAB Function  Commented=on  TreatAsAtomicUnit=on
  pid3 : MATLAB Function  Commented=on  TreatAsAtomicUnit=on
  期望横摆力矩计算 : MATLAB Function  TreatAsAtomicUnit=on
  转动惯量 : Constant  Value=145
  阿克曼转向 : MATLAB Function  TreatAsAtomicUnit=on
  M : Outport
  wires:
  Product/1 -> Sum/2
  MATLAB Function/1(y) -> 期望横摆力矩计算/1(delta)
  期望横摆力矩计算/1(Mz) -> Sum/1
  Data Store Read1/1 -> 阿克曼转向/1(v), 期望横摆力矩计算/2(Vx)
  转动惯量/1 -> Product/1, LQR差速/3(J)
  Data Store Read/1 -> MATLAB Function/1(u)
  Sum/1 -> LQR差速/1(yaw_error)
  Data Store Read3/1 -> Product/2, LQR差速/2(yaw_rate)
  阿克曼转向/3(wrl) -> Data Store Write3/1
  Data Store Read4/1 -> pid/1(v)
  Data Store Read7/1 -> pid3/1(v)
  阿克曼转向/2(wfr) -> Data Store Write2/1
  Data Store Read5/1 -> pid1/1(v)
  Data Store Read2/1 -> 阿克曼转向/2(a), 期望横摆力矩计算/3(ax)
  阿克曼转向/1(wfl) -> Data Store Write1/1
  Data Store Read6/1 -> pid2/1(v)
  阿克曼转向/4(wrr) -> Data Store Write4/1
  Data Store Read8/1 -> 阿克曼转向/3(angle)
  LQR差速/1(M) -> M/1

== system ultra/run/ctrl/Subsystem1/control_strategy/限滑/MPC ==
  右后in : Inport
  左后in : Inport  Port=2
  右前in : Inport  Port=3
  左前in : Inport  Port=4
  MPC : Subsystem
  右后 : Outport
  左后 : Outport  Port=2
  右前 : Outport  Port=3
  左前 : Outport  Port=4
  wires:
  右后in/1 -> MPC/1(U_init)
  左后in/1 -> MPC/2(U_init1)
  右前in/1 -> MPC/3(U_init2)
  左前in/1 -> MPC/4(U_init3)
  MPC/1(右后) -> 右后/1
  MPC/2(左后) -> 左后/1
  MPC/3(右前) -> 右前/1
  MPC/4(左前) -> 左前/1

== system ultra/run/ctrl/Subsystem1/control_strategy/限滑/PID限滑 ==
  u : Inport
  Constant{,1..3} (4 alike) : Constant  Value=0.9
  Data Store Read : DataStoreRead  DataStoreName=slipyouhou
  Data Store Read1 : DataStoreRead  DataStoreName=slipyuoqian
  Data Store Read2 : DataStoreRead  DataStoreName=slipzuohou
  Data Store Read3 : DataStoreRead  DataStoreName=slipzuoqian
  Data Store Write : DataStoreWrite  DataStoreName=brake_slipyouhou
  Data Store Write1 : DataStoreWrite  DataStoreName=brake_slipzuohou
  Data Store Write2 : DataStoreWrite  DataStoreName=brake_slipzuoqian
  Data Store Write3 : DataStoreWrite  DataStoreName=brake_slipyouqian
  pid限滑与ABS : MATLAB Function  TreatAsAtomicUnit=on
  pid限滑与ABS1 : MATLAB Function  TreatAsAtomicUnit=on
  pid限滑与ABS2 : MATLAB Function  TreatAsAtomicUnit=on
  pid限滑与ABS3 : MATLAB Function  TreatAsAtomicUnit=on
  计算油压 : MATLAB Function  TreatAsAtomicUnit=on
  throttle_youhou : Outport
  throttle_youqian : Outport  Port=2
  throttle_zuohou : Outport  Port=3
  throttle_zuoqian : Outport  Port=4
  wires:
  Data Store Read/1 -> pid限滑与ABS/1(slip)
  Constant/1 -> pid限滑与ABS/2(slip_ratio_limit)
  Data Store Read2/1 -> pid限滑与ABS2/1(slip)
  Constant1/1 -> pid限滑与ABS1/2(slip_ratio_limit)
  Data Store Read3/1 -> pid限滑与ABS3/1(slip)
  pid限滑与ABS/1(throttle) -> throttle_youhou/1
  Constant3/1 -> pid限滑与ABS3/2(slip_ratio_limit)
  Data Store Read1/1 -> pid限滑与ABS1/1(slip)
  Constant2/1 -> pid限滑与ABS2/2(slip_ratio_limit)
  pid限滑与ABS3/1(throttle) -> throttle_zuoqian/1
  pid限滑与ABS1/1(throttle) -> throttle_youqian/1
  pid限滑与ABS2/1(throttle) -> throttle_zuohou/1
  pid限滑与ABS3/2(brake) -> 计算油压/1(y1)
  pid限滑与ABS1/2(brake) -> 计算油压/2(y2)
  pid限滑与ABS2/2(brake) -> 计算油压/3(y3)
  pid限滑与ABS/2(brake) -> 计算油压/4(y4)
  计算油压/4(p4) -> Data Store Write/1
  计算油压/1(p1) -> Data Store Write2/1
  计算油压/2(p2) -> Data Store Write3/1
  计算油压/3(p3) -> Data Store Write1/1
  u/1 -> pid限滑与ABS3/3(u), pid限滑与ABS2/3(u), pid限滑与ABS1/3(u), pid限滑与ABS/3(u)

== system ultra/run/ctrl/Subsystem1/control_strategy/限滑/Subsystem1 ==
  TP : Inport
  右后 : Inport  Port=2
  throttle_youhou : Inport  Port=3
  In4 : Inport  Port=4
  右前 : Inport  Port=5
  throttle_youqian : Inport  Port=6
  u : Inport  Port=7
  mpc : Inport  Port=8
  pid : Inport  Port=9
  In7 : Inport  Port=10
  左前 : Inport  Port=11
  throttle_zuoqian : Inport  Port=12
  Data Store Read : DataStoreRead  DataStoreName=slipyouhou
  Data Store Read1 : DataStoreRead  DataStoreName=slipyuoqian
  Data Store Read2 : DataStoreRead  DataStoreName=slipzuohou
  Data Store Read3 : DataStoreRead  DataStoreName=slipzuoqian
  Data Store Read4 : DataStoreRead  DataStoreName=match_model
  MATLAB Function2 : MATLAB Function  TreatAsAtomicUnit=on
  MATLAB Function3 : MATLAB Function  TreatAsAtomicUnit=on
  MATLAB Function4 : MATLAB Function  TreatAsAtomicUnit=on
  MATLAB Function5 : MATLAB Function  TreatAsAtomicUnit=on
  youhou : Outport
  youqian : Outport  Port=2
  zuohou : Outport  Port=3
  zuoqian : Outport  Port=4
  wires:
  pid/1 -> MATLAB Function5/3(pid)
  mpc/1 -> MATLAB Function5/2(mpc)
  u/1 -> MATLAB Function5/1(u)
  In4/1 -> MATLAB Function4/1(u)
  右前/1 -> MATLAB Function4/2(mpc)
  throttle_youqian/1 -> MATLAB Function4/3(pid)
  throttle_youhou/1 -> MATLAB Function3/3(pid)
  右后/1 -> MATLAB Function3/2(mpc)
  TP/1 -> MATLAB Function3/1(u)
  throttle_zuoqian/1 -> MATLAB Function2/3(pid)
  左前/1 -> MATLAB Function2/2(mpc)
  In7/1 -> MATLAB Function2/1(u)
  Data Store Read/1 -> MATLAB Function3/4(slip)
  Data Store Read1/1 -> MATLAB Function4/4(slip)
  Data Store Read2/1 -> MATLAB Function5/4(slip)
  Data Store Read3/1 -> MATLAB Function2/4(slip)
  MATLAB Function3/1(y) -> youhou/1
  MATLAB Function2/1(y) -> zuoqian/1
  MATLAB Function5/1(y) -> zuohou/1
  MATLAB Function4/1(y) -> youqian/1
  Data Store Read4/1 -> MATLAB Function2/5(model), MATLAB Function5/5(model), MATLAB Function4/5(model), MATLAB Function3/5(model)

== system ultra/run/analog_input/无人意图转译/无人/Subsystem1/Desired/Subsystem ==
  y : Inport
  Delay : Delay  DelayLength=1
  Delay1 : Delay
  Delay2 : Delay  DelayLength=3
  Delay3 : Delay  DelayLength=4
  u2 : Outport
  u3 : Outport  Port=2
  u4 : Outport  Port=3
  u5 : Outport  Port=4
  wires:
  y/1 -> Delay3/1, Delay2/1, Delay1/1, Delay/1
  Delay/1 -> u2/1
  Delay1/1 -> u3/1
  Delay3/1 -> u5/1
  Delay2/1 -> u4/1

== system ultra/run/analog_input/无人意图转译/无人/Subsystem1/Desired/Subsystem1 ==
  y : Inport
  Delay : Delay  DelayLength=1
  Delay1 : Delay
  Delay2 : Delay  DelayLength=3
  Delay3 : Delay  DelayLength=4
  u2 : Outport
  u3 : Outport  Port=2
  u4 : Outport  Port=3
  u5 : Outport  Port=4
  wires:
  y/1 -> Delay3/1, Delay2/1, Delay1/1, Delay/1
  Delay/1 -> u2/1
  Delay1/1 -> u3/1
  Delay3/1 -> u5/1
  Delay2/1 -> u4/1

== system ultra/run/analog_input/无人意图转译/无人/Subsystem1/Subsystem/pid_function ==
  u : Inport
  期望加速度（负值） : Inport  Port=2
  Abs1 : Abs  Commented=on
  Gain : Gain  Commented=on
  Gain2 : Gain  Commented=on
  Subsystem : Subsystem  Commented=on
  integral : MATLAB Function  TreatAsAtomicUnit=on
  output : Outport
  wires:
  integral/1(output) -> output/1
  Gain/1 -> Abs1/1
  u/1 -> integral/1(u)
  Gain2/1 -> Subsystem/1(In1)
  期望加速度（负值）/1 -> integral/2(a)

== system ultra/run/ctrl/Subsystem1/control_strategy/限滑/MPC/MPC ==
  U_init : Inport
  U_init1 : Inport  Port=2
  U_init2 : Inport  Port=3
  U_init3 : Inport  Port=4
  Data Store Read : DataStoreRead  DataStoreName=slipyouhou
  Data Store Read1 : DataStoreRead  DataStoreName=slipzuohou
  Data Store Read2 : DataStoreRead  DataStoreName=slipyuoqian
  Data Store Read3 : DataStoreRead  DataStoreName=slipzuoqian
  MATLAB Function : MATLAB Function  TreatAsAtomicUnit=on
  MATLAB Function1 : MATLAB Function  TreatAsAtomicUnit=on
  MATLAB Function2 : MATLAB Function  TreatAsAtomicUnit=on
  MATLAB Function3 : MATLAB Function  TreatAsAtomicUnit=on
  MPC右前 : Subsystem
  MPC右后 : Subsystem
  MPC左前 : Subsystem
  MPC左后 : Subsystem
  右后 : Outport
  左后 : Outport  Port=2
  右前 : Outport  Port=3
  左前 : Outport  Port=4
  wires:
  MPC右前/1(右前) -> 右前/1
  MPC左前/1(左前) -> 左前/1
  MPC右后/1(右后) -> 右后/1
  U_init3/1 -> MPC左前/1(U_init)
  MPC左后/1(左后) -> 左后/1
  U_init1/1 -> MPC左后/1(U_init)
  U_init2/1 -> MPC右前/1(U_init)
  U_init/1 -> MPC右后/1(U_init)
  Data Store Read/1 -> MATLAB Function/1(u)
  MATLAB Function/1(y) -> MPC右后/Enable
  Data Store Read1/1 -> MATLAB Function1/1(u)
  MATLAB Function1/1(y) -> MPC左后/Enable
  Data Store Read2/1 -> MATLAB Function2/1(u)
  MATLAB Function2/1(y) -> MPC右前/Enable
  Data Store Read3/1 -> MATLAB Function3/1(u)
  MATLAB Function3/1(y) -> MPC左前/Enable

== system ultra/run/analog_input/无人意图转译/无人/Subsystem1/Subsystem/pid_function/Subsystem ==
  In1 : Inport
  Constant1 : Constant  Value=0.02
  Delay1 : Delay  DelayLength=1
  Divide1 : Product  Inputs=*/
  Sum4 : Sum  Inputs=|+-
  Out1 : Outport
  wires:
  Divide1/1 -> Out1/1
  Constant1/1 -> Divide1/2
  Sum4/1 -> Divide1/1
  Delay1/1 -> Sum4/2
  In1/1 -> Sum4/1, Delay1/1

== system ultra/run/ctrl/Subsystem1/control_strategy/限滑/MPC/MPC/MPC右前 ==
  U_init : Inport
  Enable : EnablePort
  Constant : Constant  Value=0.17
  Data Store Read : DataStoreRead  DataStoreName=slipyuoqian
  MPC_function : MATLAB Function  TreatAsAtomicUnit=on
  Sum : Sum  Inputs=|+-
  右前 : Outport
  wires:
  Data Store Read/1 -> Sum/1
  Constant/1 -> Sum/2
  MPC_function/1(u_k) -> 右前/1
  Sum/1 -> MPC_function/1(x_k)
  U_init/1 -> MPC_function/2(U_init)

== system ultra/run/ctrl/Subsystem1/control_strategy/限滑/MPC/MPC/MPC右后 ==
  U_init : Inport
  Enable : EnablePort
  Constant : Constant  Value=0.17
  Data Store Read : DataStoreRead  DataStoreName=slipyouhou
  MPC_function : MATLAB Function  TreatAsAtomicUnit=on
  Sum : Sum  Inputs=|+-
  右后 : Outport
  wires:
  Data Store Read/1 -> Sum/1
  Constant/1 -> Sum/2
  MPC_function/1(u_k) -> 右后/1
  Sum/1 -> MPC_function/1(x_k)
  U_init/1 -> MPC_function/2(U_init)

== system ultra/run/ctrl/Subsystem1/control_strategy/限滑/MPC/MPC/MPC左前 ==
  U_init : Inport
  Enable : EnablePort
  Constant : Constant  Value=0.17
  Data Store Read : DataStoreRead  DataStoreName=slipzuoqian
  MPC_function : MATLAB Function  TreatAsAtomicUnit=on
  Sum : Sum  Inputs=|+-
  左前 : Outport
  wires:
  Data Store Read/1 -> Sum/1
  Constant/1 -> Sum/2
  MPC_function/1(u_k) -> 左前/1
  Sum/1 -> MPC_function/1(x_k)
  U_init/1 -> MPC_function/2(U_init)

== system ultra/run/ctrl/Subsystem1/control_strategy/限滑/MPC/MPC/MPC左后 ==
  U_init : Inport
  Enable : EnablePort
  Constant : Constant  Value=0.17
  Data Store Read : DataStoreRead  DataStoreName=slipzuohou
  MPC_function : MATLAB Function  TreatAsAtomicUnit=on
  Sum : Sum  Inputs=|+-
  左后 : Outport
  wires:
  Data Store Read/1 -> Sum/1
  Constant/1 -> Sum/2
  MPC_function/1(u_k) -> 左后/1
  Sum/1 -> MPC_function/1(x_k)
  U_init/1 -> MPC_function/2(U_init)

== matlab function ultra/TX控制器/速度/188右后/MATLAB Function3 ==
  data: v input; y output; angle input; vz input; model input
function y = fcn(v, angle,vz,model)
if (angle>3||angle<-3)&&model==3%4650000,4870000,4741002
    y=vz*594.06;
else
    y = v;
end

== matlab function ultra/TX控制器/速度/189左后/MATLAB Function3 ==
  data: v input; y output; angle input; vz input; model input
function y = fcn(v, angle, vz,model)
if (angle>3||angle<-3)&&model==3%4650000,4870000,4741002
    y=vz*594.06;
else
    y = v;
end

== matlab function ultra/无人TX/转向换算/Subsystem/MATLAB Function1 ==
  data: u input; y output
function y = fcn(u)

y = (u-2.846e+04)/3255;

== matlab function ultra/TX控制器/Subsystem1/MATLAB Function2 ==
  data: anglenb input; youqianvvv output; v input; zuoqianvvv output; youhouvvv output; zuohouvvv output; model input; k input
function [youqianvvv,zuoqianvvv,youhouvvv,zuohouvvv] = fcn(anglenb,v,model,k)

angle=anglenb*pi/180;
if model==3
    k=k+0.5;
    if angle>0
        zuohouvvv=v*(1.53/(k*angle)+1.16)/(1.53/(k*angle)+0.58);
        youhouvvv=v*(1.53/(k*angle))/(1.53/(k*angle)+0.58);
        zuoqianvvv=v*(1.53/(k*angle)+1.18)/(1.53/(k*angle)+0.59);
        youqianvvv=v*(1.53/(k*angle))/(1.53/(k*angle)+0.59);
    else
        youhouvvv=v*(1.53/(-k*angle)+1.16)/(-1.53/(k*angle)+0.58);
        zuohouvvv=v*(-1.53/(k*angle))/(-1.53/(k*angle)+0.58);
        youqianvvv=v*(-1.53/(k*angle)+1.18)/(-1.53/(k*angle)+0.59);
        zuoqianvvv=v*(-1.53/(k*angle))/(-1.53/(k*angle)+0.59);
    end
else
    zuohouvvv=v;
    youhouvvv=v;
    zuoqianvvv=v;
    youqianvvv=v;
end
